simulink model "InjCrv_PoI2Set"  (R2016b)
settings: configuration reference "CodeGenConfigSet" (kept outside this file)
values from neighbouring files (symbols this model uses):
  InjCrv_facPoI2EffEOM_MAP = Calibration.Parameter    [init_InjCrv_PoI2Set.m]
  InjCrv_facPoI2EffEOM_MAPX = Calibration.Parameter    [init_InjCrv_PoI2Set.m]
  InjCrv_facPoI2EffEOM_MAPY = Calibration.Parameter    [init_InjCrv_PoI2Set.m]
  InjCrv_phiPoI2BasEOM_MAP = Calibration.Parameter    [init_InjCrv_PoI2Set.m]
  InjCrv_phiPoI2BasEOM_MAPX = Calibration.Parameter    [init_InjCrv_PoI2Set.m]
  InjCrv_phiPoI2BasEOM_MAPY = Calibration.Parameter    [init_InjCrv_PoI2Set.m]
  InjCrv_qPoI2BasEOM_MAP = Calibration.Parameter    [init_InjCrv_PoI2Set.m]
  InjCrv_qPoI2BasEOM_MAPX = Calibration.Parameter    [init_InjCrv_PoI2Set.m]
  InjCrv_qPoI2BasEOM_MAPY = Calibration.Parameter    [init_InjCrv_PoI2Set.m]
  InjCrv_tiPoI2BasEOM_MAP = Calibration.Parameter    [init_InjCrv_PoI2Set.m]
  InjCrv_tiPoI2BasEOM_MAPX = Calibration.Parameter    [init_InjCrv_PoI2Set.m]
  InjCrv_tiPoI2BasEOM_MAPY = Calibration.Parameter    [init_InjCrv_PoI2Set.m]
settings Model: Creator=Administrator  LastModifiedBy=wangrui
settings ConfigSetRef: SourceLocation=Base Workspace

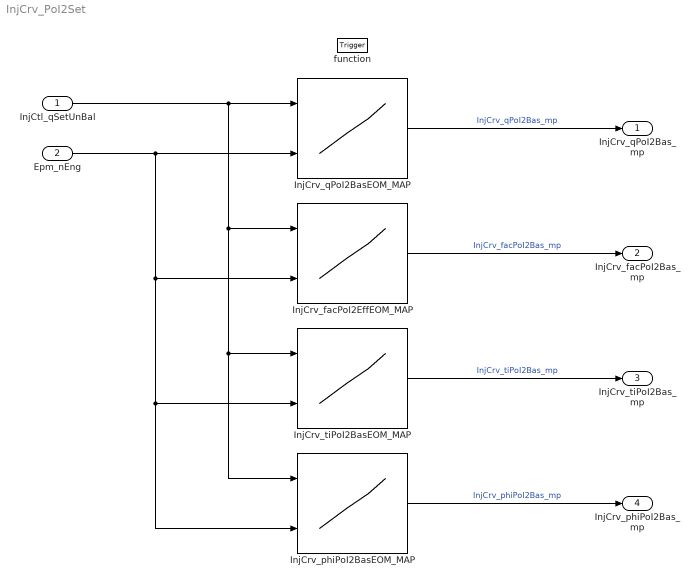
== system InjCrv_PoI2Set ==
  InjCtl_qSetUnBal : Inport  Tag=mg/hub  Description=Current injection quantity  OutMin=-319  OutMax=319  OutDataTypeStr=FuelMass_mg_hub
  Epm_nEng : Inport  Tag=rpm  Description=Engine speed  Port=2  OutMin=0  OutMax=6000  OutDataTypeStr=EngSpeed_rpm
  function : TriggerPort  TriggerType=function-call  VariantControl=Variant
  InjCrv_facPoI2EffEOM_MAP : Lookup_n-D  BreakpointsForDimension1=InjCrv_facPoI2EffEOM_MAPY  BreakpointsForDimension2=InjCrv_facPoI2EffEOM_MAPX  IndexSearchMethod=Linear search  BeginIndexSearchUsingPreviousIndexResult=on  Table=InjCrv_facPoI2EffEOM_MAP  ExtrapMethod=Clip  UseLastTableValue=on  InternalRulePriority=Speed  OutDataTypeStr=Inherit: Inherit via back propagation  RndMeth=Simplest  SaturateOnIntegerOverflow=on
  InjCrv_phiPoI2BasEOM_MAP : Lookup_n-D  BreakpointsForDimension1=InjCrv_phiPoI2BasEOM_MAPY  BreakpointsForDimension2=InjCrv_phiPoI2BasEOM_MAPX  IndexSearchMethod=Linear search  BeginIndexSearchUsingPreviousIndexResult=on  Table=InjCrv_phiPoI2BasEOM_MAP  ExtrapMethod=Clip  UseLastTableValue=on  InternalRulePriority=Speed  OutDataTypeStr=Inherit: Inherit via back propagation  RndMeth=Simplest  SaturateOnIntegerOverflow=on
  InjCrv_qPoI2BasEOM_MAP : Lookup_n-D  BreakpointsForDimension1=InjCrv_qPoI2BasEOM_MAPY  BreakpointsForDimension2=InjCrv_qPoI2BasEOM_MAPX  IndexSearchMethod=Linear search  BeginIndexSearchUsingPreviousIndexResult=on  Table=InjCrv_qPoI2BasEOM_MAP  ExtrapMethod=Clip  UseLastTableValue=on  InternalRulePriority=Speed  OutDataTypeStr=Inherit: Inherit via back propagation  RndMeth=Simplest  SaturateOnIntegerOverflow=on
  InjCrv_tiPoI2BasEOM_MAP : Lookup_n-D  BreakpointsForDimension1=InjCrv_tiPoI2BasEOM_MAPY  BreakpointsForDimension2=InjCrv_tiPoI2BasEOM_MAPX  IndexSearchMethod=Linear search  BeginIndexSearchUsingPreviousIndexResult=on  Table=InjCrv_tiPoI2BasEOM_MAP  ExtrapMethod=Clip  UseLastTableValue=on  InternalRulePriority=Speed  OutDataTypeStr=Inherit: Inherit via back propagation  RndMeth=Simplest  SaturateOnIntegerOverflow=on
  InjCrv_qPoI2Bas_mp : Outport  Tag=mg/hub  Description=PoI2 base quantity for injection  OutMin=-319  OutMax=319  OutDataTypeStr=FuelMass_mg_hub
  InjCrv_facPoI2Bas_mp : Outport  Description=PoI2 base Efficiency factor  Port=2  OutMin=-10  OutMax=10  OutDataTypeStr=Factor
  InjCrv_tiPoI2Bas_mp : Outport  Tag=us  Description=PoI2 base start of energizing of time  Port=3  OutMin=-13107  OutMax=13106  OutDataTypeStr=InjTime_us
  InjCrv_phiPoI2Bas_mp : Outport  Tag=CA  Description=PoI2 base start of energizing of angle  Port=4  OutMin=-719  OutMax=719  OutDataTypeStr=Angle_CA
  wires:
  InjCtl_qSetUnBal/1 -> InjCrv_phiPoI2BasEOM_MAP/1, InjCrv_tiPoI2BasEOM_MAP/1, InjCrv_facPoI2EffEOM_MAP/1, InjCrv_qPoI2BasEOM_MAP/1
  Epm_nEng/1 -> InjCrv_phiPoI2BasEOM_MAP/2, InjCrv_tiPoI2BasEOM_MAP/2, InjCrv_facPoI2EffEOM_MAP/2, InjCrv_qPoI2BasEOM_MAP/2
  InjCrv_qPoI2BasEOM_MAP/1 -> InjCrv_qPoI2Bas_mp/1  "InjCrv_qPoI2Bas_mp"
  InjCrv_facPoI2EffEOM_MAP/1 -> InjCrv_facPoI2Bas_mp/1  "InjCrv_facPoI2Bas_mp"
  InjCrv_tiPoI2BasEOM_MAP/1 -> InjCrv_tiPoI2Bas_mp/1  "InjCrv_tiPoI2Bas_mp"
  InjCrv_phiPoI2BasEOM_MAP/1 -> InjCrv_phiPoI2Bas_mp/1  "InjCrv_phiPoI2Bas_mp"
